simulink model "lab4"  (R2022b)
settings: Solver=FixedStepAuto  StartTime=0.0  StopTime=10  FixedStep=0.0001  RelTol=1e-3
undefined symbols (not defined in the file): g, l
settings Model: Creator=dambi  LastModifiedBy=dambi

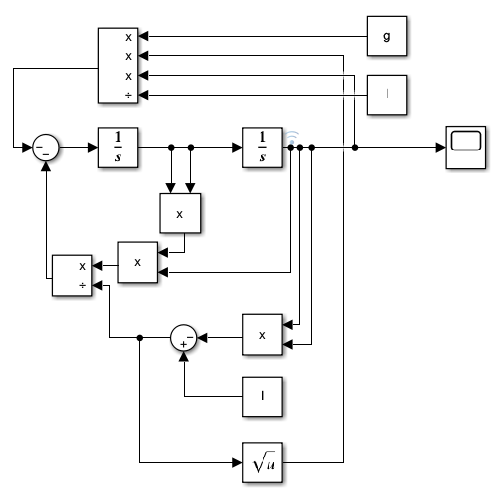
[thumbnail: Simulink's stored preview of the top-level diagram]
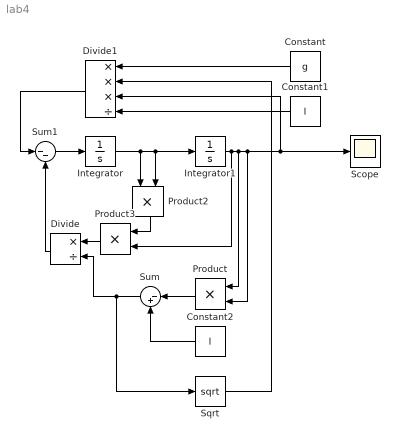
== system lab4 ==
  Constant : Constant  Value=g
  Constant1 : Constant  Value=l
  Constant2 : Constant  Value=l
  Divide : Product  Inputs=*/
  Divide1 : Product  Inputs=***/
  Integrator : Integrator  InitialCondition=1
  Integrator1 : Integrator  InitialCondition=1
  Product : Product
  Product2 : Product
  Product3 : Product
  Scope : Scope
  Sqrt : Sqrt
  Sum : Sum  Inputs=|-+
  Sum1 : Sum  Inputs=|--
  wires:
  Sum1/1 -> Integrator/1
  Product2/1 -> Product3/1
  Integrator/1 -> Integrator1/1, Product2/2, Product2/1
  Constant2/1 -> Sum/2
  Product/1 -> Sum/1
  Product3/1 -> Divide/1
  Divide/1 -> Sum1/2
  Sum/1 -> Sqrt/1, Divide/2
  Integrator1/1 -> Scope/1, Divide1/3, Product/2, Product/1, Product3/2
  Constant/1 -> Divide1/1
  Constant1/1 -> Divide1/4
  Sqrt/1 -> Divide1/2
  Divide1/1 -> Sum1/1
